simulink model "model_test_pi"  (R2024b)
settings: Solver=VariableStepAuto  StartTime=0.0  StopTime=10.0  RelTol=1e-3
libraries: simulink x2
settings Model: Creator=mehmetcanevi  LastModifiedBy=mehmetcanevi

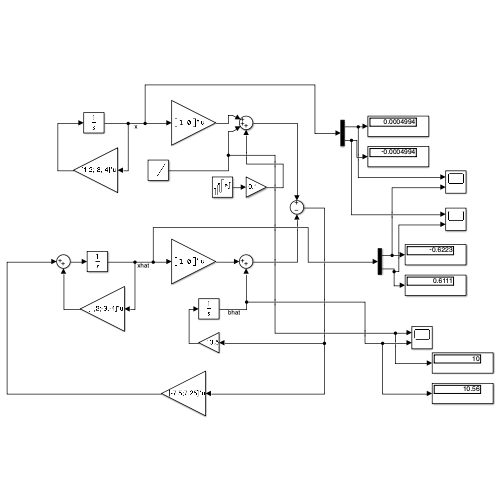
[thumbnail: Simulink's stored preview of the top-level diagram]
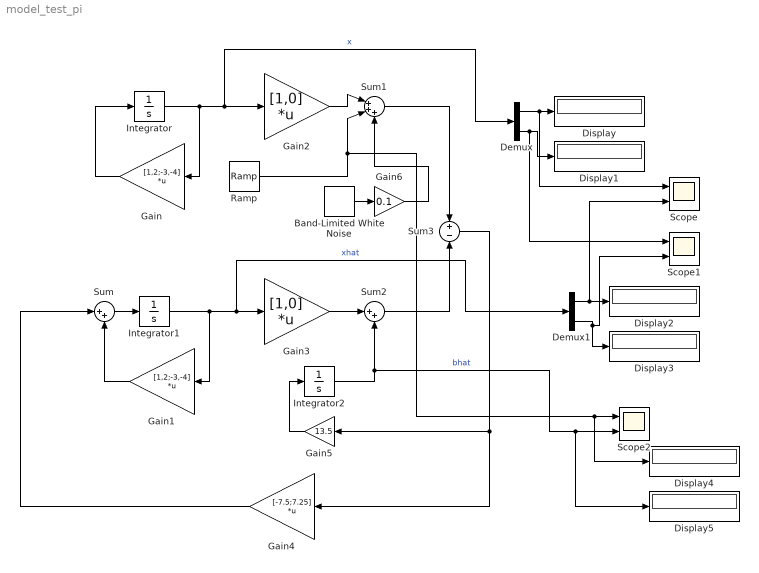
== system model_test_pi ==
  Band-Limited White Noise : simulink/Sources/Band-Limited White Noise  Cov=[0.1]  Ts=0.1  seed=[23341]
  Demux : Demux  Outputs=2
  Demux1 : Demux  Outputs=2
  Display{,1..5} (6 alike) : Display
  Gain : Gain  Gain=[1,2;-3,-4]  Multiplication=Matrix(K*u)
  Gain1 : Gain  Gain=[1,2;-3,-4]  Multiplication=Matrix(K*u)
  Gain2 : Gain  Gain=[1,0]  Multiplication=Matrix(K*u)
  Gain3 : Gain  Gain=[1,0]  Multiplication=Matrix(K*u)
  Gain4 : Gain  Gain=[-7.5;7.25]  Multiplication=Matrix(K*u)
  Gain5 : Gain  Gain=13.5
  Gain6 : Gain  Gain=0.1
  Integrator : Integrator  InitialCondition=[3;1]
  Integrator1 : Integrator
  Integrator2 : Integrator
  Ramp : simulink/Sources/Ramp  slope=1  start=0  InitialOutput=0
  Scope : Scope  NumInputPorts=2
  Scope1 : Scope  NumInputPorts=2
  Scope2 : Scope  NumInputPorts=2
  Sum : Sum  Inputs=|++
  Sum1 : Sum  Inputs=|+++
  Sum2 : Sum  Inputs=|++
  Sum3 : Sum  Inputs=+-
  wires:
  Gain/1 -> Integrator/1
  Integrator/1 -> Demux/1, Gain2/1, Gain/1  "x"
  Sum/1 -> Integrator1/1
  Gain1/1 -> Sum/2
  Gain2/1 -> Sum1/1
  Ramp/1 -> Display4/1, Scope2/1, Sum1/2
  Gain3/1 -> Sum2/1
  Sum1/1 -> Sum3/1
  Sum2/1 -> Sum3/2
  Sum3/1 -> Gain5/1, Gain4/1
  Gain4/1 -> Sum/1
  Demux/1 -> Scope/1, Display/1
  Demux/2 -> Scope1/1, Display1/1
  Demux1/2 -> Scope1/2, Display3/1
  Integrator1/1 -> Demux1/1, Gain3/1, Gain1/1  "xhat"
  Demux1/1 -> Scope/2, Display2/1
  Gain5/1 -> Integrator2/1
  Integrator2/1 -> Sum2/2, Display5/1, Scope2/2  "bhat"
  Band-Limited White Noise/1 -> Gain6/1
  Gain6/1 -> Sum1/3
